simulink model "toFWDEuler"  (Simulink 7.9)
settings: Solver=ode3  StartTime=0.0  StopTime=10.0  FixedStep=0.001  RelTol=1e-3
undefined symbols (not defined in the file or in its folder): ARULE, TransformationLib
libraries: Post_CommonlyUsedBlocks x5, Pre_CommonlyUsedBlocks x3
settings Model: Creator=denil  LastModifiedBy=jdenil

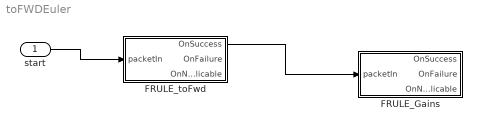
== system toFWDEuler ==
  start : Inport
  FRULE_Gains : Subsystem  AncestorBlock=TransformationLib/ARULE
  FRULE_toFwd : Subsystem  AncestorBlock=TransformationLib/ARULE
  wires:
  FRULE_toFwd/1(OnSuccess) -> FRULE_Gains/1(packetIn)
  start/1 -> FRULE_toFwd/1(packetIn)

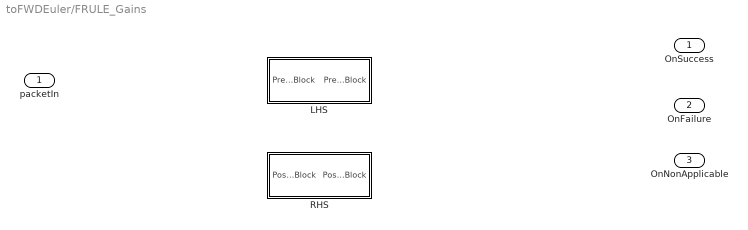
== system toFWDEuler/FRULE_Gains ==
  packetIn : Inport
  LHS : Subsystem
  RHS : Subsystem
  OnSuccess : Outport
  OnFailure : Outport  Port=2
  OnNonApplicable : Outport  Port=3

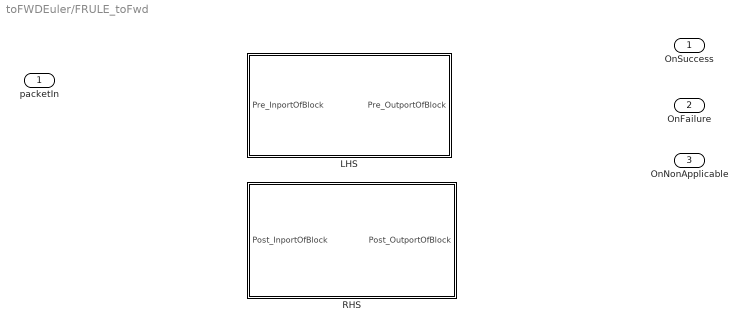
== system toFWDEuler/FRULE_toFwd ==
  packetIn : Inport
  LHS : Subsystem
  RHS : Subsystem
  OnSuccess : Outport
  OnFailure : Outport  Port=2
  OnNonApplicable : Outport  Port=3

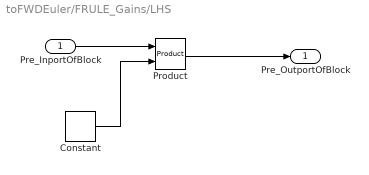
== system toFWDEuler/FRULE_Gains/LHS ==
  Pre_InportOfBlock : Inport  LibraryBlock=Pre_CommonlyUsedBlocks/Pre_InportOfBlock  pre_label=0
      settings: AttributesFormatString=%<pre_label>
  Constant : Pre_CommonlyUsedBlocks/Constant  pre_label=1  pre_value=return True  pre_Name=return True  pre_Position=return True
      settings: AttributesFormatString=%<pre_label>
  Product : Pre_CommonlyUsedBlocks/Product  pre_label=2  pre_Name=return True  pre_Position=return True
      settings: AttributesFormatString=%<pre_label>
  Pre_OutportOfBlock : Outport  LibraryBlock=Pre_CommonlyUsedBlocks/Pre_OutportOfBlock  pre_label=4
      settings: AttributesFormatString=%<pre_label>
  wires:
  Pre_InportOfBlock/1 -> Product/1
  Constant/1 -> Product/2
  Product/1 -> Pre_OutportOfBlock/1

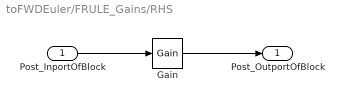
== system toFWDEuler/FRULE_Gains/RHS ==
  Post_InportOfBlock : Inport  LibraryBlock=Post_CommonlyUsedBlocks/Post_InportOfBlock  post_label=0
      settings: AttributesFormatString=%<post_label>
  Gain : Post_CommonlyUsedBlocks/Gain  post_label=5  post_gain=return PreNode('1')['value']  post_Name=return PreNode('1')['Name']+'Gain'  post_Position=return PreNode('1')['Position']
      settings: AttributesFormatString=%<post_label>
  Post_OutportOfBlock : Outport  LibraryBlock=Post_CommonlyUsedBlocks/Post_OutportOfBlock  post_label=4
      settings: AttributesFormatString=%<post_label>
  wires:
  Post_InportOfBlock/1 -> Gain/1
  Gain/1 -> Post_OutportOfBlock/1

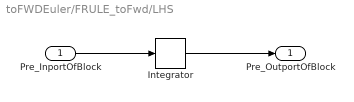
== system toFWDEuler/FRULE_toFwd/LHS ==
  Pre_InportOfBlock : Inport  LibraryBlock=Pre_CommonlyUsedBlocks/Pre_InportOfBlock  pre_label=0
      settings: AttributesFormatString=%<pre_label>
  Integrator : Pre_CommonlyUsedBlocks/Integrator  pre_label=1  pre_initial=return True  pre_Name=return True  pre_Position=return True
      settings: AttributesFormatString=%<pre_label>
  Pre_OutportOfBlock : Outport  LibraryBlock=Pre_CommonlyUsedBlocks/Pre_OutportOfBlock  pre_label=2
      settings: AttributesFormatString=%<pre_label>
  wires:
  Pre_InportOfBlock/1 -> Integrator/1
  Integrator/1 -> Pre_OutportOfBlock/1

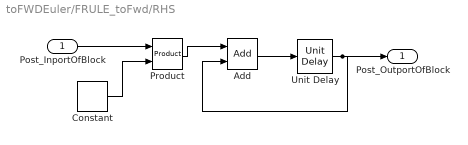
== system toFWDEuler/FRULE_toFwd/RHS ==
  Post_InportOfBlock : Inport  LibraryBlock=Post_CommonlyUsedBlocks/Post_InportOfBlock  post_label=0
      settings: AttributesFormatString=%<post_label>
  Add : Post_CommonlyUsedBlocks/Add  post_label=4  post_Name=return PreNode('1')['Name']+'Add'  post_Position=return PreNode('1')['Position']
      settings: AttributesFormatString=%<post_label>
  Constant : Post_CommonlyUsedBlocks/Constant  post_label=6  post_value=return 0.001  post_Name=return PreNode('1')['Name']+'gainconst'  post_Position=return PreNode('1')['Position']
      settings: AttributesFormatString=%<post_label>
  Product : Post_CommonlyUsedBlocks/Product  post_label=3  post_Name=return PreNode('1')['Name']+'Product'  post_Position=return PreNode('1')['Position']
      settings: AttributesFormatString=%<post_label>
  Unit Delay : Post_CommonlyUsedBlocks/Unit Delay  post_label=5  post_initial=return PreNode('1')['InitialCondition']  post_Name=return PreNode('1')['Name']+'Delay'  post_Position=return PreNode('1')['Position']
      settings: AttributesFormatString=%<post_label>
  Post_OutportOfBlock : Outport  LibraryBlock=Post_CommonlyUsedBlocks/Post_OutportOfBlock  post_label=2
      settings: AttributesFormatString=%<post_label>
  wires:
  Post_InportOfBlock/1 -> Product/1
  Product/1 -> Add/1
  Add/1 -> Unit Delay/1
  Unit Delay/1 -> Post_OutportOfBlock/1, Add/2
  Constant/1 -> Product/2
